simulink model "BuckRegulatorMicrocontroller"  (R2023b)
settings: Solver=FixedStepAuto  StartTime=0.0  StopTime=10.0  RelTol=1e-3  EnableMultiTasking=on
model workspace (MAT data in the model file):
  C = Simulink.Parameter
  C.Value = 0.001
  C.Description = 'Output capacitor'
  C.DataType = 'auto'
  C.DocUnits = 'F'
  C.Complexity = 'real'
  C.Dimensions = [1 1]
  L = Simulink.Parameter
  L.Value = 0.001
  L.Description = 'Buck inductor value'
  L.DataType = 'auto'
  L.DocUnits = 'H'
  L.Complexity = 'real'
  L.Dimensions = [1 1]
  R = Simulink.Parameter
  R.Value = 15
  R.Description = 'Load resistor'
  R.DataType = 'auto'
  R.DocUnits = 'Ω'
  R.Complexity = 'real'
  R.Dimensions = [1 1]
  Vs = Simulink.Parameter
  Vs.Value = 10
  Vs.Description = 'Converter input voltage'
  Vs.DataType = 'auto'
  Vs.DocUnits = 'V'
  Vs.Complexity = 'real'
  Vs.Dimensions = [1 1]
settings Model: Creator=Mazen  LastModifiedBy=Mazen
settings OptimizationCC: DefaultParameterBehavior=Inlined  UseDivisionForNetSlopeComputation=on  GainParamInheritBuiltInType=on  UseFloatMulNetSlope=on  InlineInvariantSignals=on  StrengthReduction=on  PassReuseOutputArgsAs=Individual arguments  ZeroExternalMemoryAtStartup=off  ZeroInternalMemoryAtStartup=off  NoFixptDivByZeroProtection=on  EfficientFloat2IntCast=on  LifeSpan=1  MaxStackSize=64  OptimizeBlockOrder=speed  OptimizationPriority=Speed  OptimizationCustomize=off  MultiThreadedLoops=on  EfficientTunableParamExpr=on
settings DebuggingCC: ParameterTunabilityLossMsg=error
settings HardwareCC: ProdBitPerPointer=32  ProdBitPerSizeT=32  ProdBitPerPtrDiffT=32  ProdLargestAtomicInteger=Long  ProdLargestAtomicFloat=Double  ProdWordSize=32  ProdHWDeviceType=ARM Compatible->ARM Cortex-M
settings SFSimCC: MATLABDynamicMemAlloc=off
settings RTWCC: Description=Embedded Coder  SystemTargetFile=ert.tlc  GenCodeOnly=on  TemplateMakefile=ert_default_tmf  Toolchain=GNU Tools for ARM Embedded Processors  BuildConfiguration=Faster Runs
settings CodeAppCC: ForceParamTrailComments=on  IgnoreCustomStorageClasses=off  OperatorAnnotations=on  SimulinkDataObjDesc=on  SFDataObjDesc=on  CustomSymbolStrGlobalVar=rt$N$M  CustomSymbolStrType=$N$M  CustomSymbolStrFcn=$N$M$F  CustomSymbolStrMacro=$N$M  InsertBlockDesc=on
settings ERTTargetCC: CodeReplacementLibrary=ARM Cortex-M  IncludeMdlTerminateFcn=off  CombineSignalStateStructs=on  SupportAbsoluteTime=off  SupportComplex=off  SupportContinuousTime=on  ExtModeTransport=3  ExtModeStaticAlloc=on  ExtModeStaticAllocSize=2048  ExtModeMexFile=ext_xcp  ExtModeIntrfLevel=Level2 - Open  InlinedParameterPlacement=NonHierarchical  ERTCustomFileTemplate=example_file_process.tlc  ERTFilePackagingFormat=CompactWithDataFile

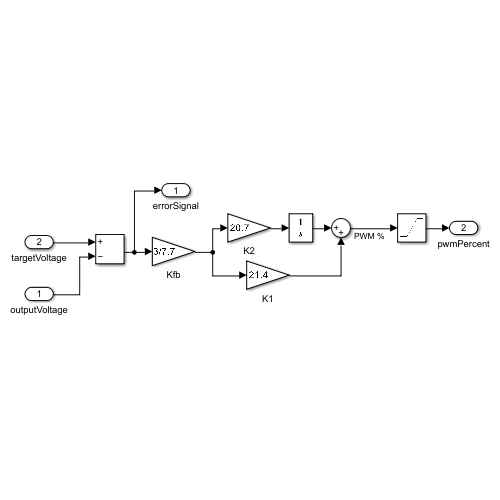
[thumbnail: Simulink's stored preview of the top-level diagram]
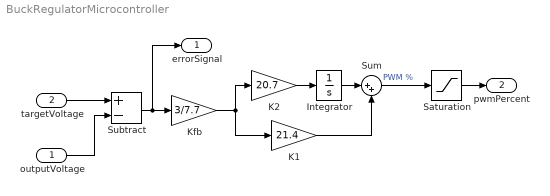
== system BuckRegulatorMicrocontroller ==
  outputVoltage : Inport
  targetVoltage : Inport  Port=2
  Integrator : Integrator
  K1 : Gain  Gain=21.4
  K2 : Gain  Gain=20.7
  Kfb : Gain  Gain=3/7.7
  Saturation : Saturate  UpperLimit=1  LowerLimit=0
  Subtract : Sum  Inputs=+-
  Sum : Sum  Inputs=|++
  errorSignal : Outport
  pwmPercent : Outport  Port=2
  wires:
  Integrator/1 -> Sum/1
  Subtract/1 -> errorSignal/1, Kfb/1
  K1/1 -> Sum/2
  Kfb/1 -> K2/1, K1/1
  Sum/1 -> Saturation/1  "PWM %"
  targetVoltage/1 -> Subtract/1
  K2/1 -> Integrator/1
  outputVoltage/1 -> Subtract/2
  Saturation/1 -> pwmPercent/1
